simulink model "OutputCalibration"  (R2024b)
settings: Solver=FixedStepAuto  StartTime=0.0  StopTime=inf  FixedStep=1/200  RelTol=1e-3  EnableMultiTasking=on
libraries: mbedblockslib x3
settings Model: ExtModeTrigDuration=10  Creator=patri  LastModifiedBy=Jaylen
settings SolverCC: AutoInsertRateTranBlk=on
settings OptimizationCC: EnhancedBackFolding=on  PassReuseOutputArgsAs=Individual arguments  ZeroExternalMemoryAtStartup=off  ZeroInternalMemoryAtStartup=off  MaxStackSize=64  OptimizeBlockOrder=speed  DifferentSizesBufferReuse=on  OptimizationCustomize=off  EfficientTunableParamExpr=on
settings DebuggingCC: ParameterTunabilityLossMsg=error
settings HardwareCC: ProdBitPerPointer=32  ProdBitPerSizeT=32  ProdBitPerPtrDiffT=32  ProdLargestAtomicInteger=Long  ProdLargestAtomicFloat=Double  ProdWordSize=32  ProdLongLongMode=on  ProdHWDeviceType=ARM Compatible->ARM Cortex-M
settings SFSimCC: MATLABDynamicMemAlloc=off
settings RTWCC: Description=Embedded Coder  SystemTargetFile=ert.tlc  HardwareBoard=STM32 Nucleo F767ZI  TemplateMakefile=ert_default_tmf  Toolchain=GNU Tools for ARM Embedded Processors
settings CodeAppCC: ForceParamTrailComments=on  IgnoreCustomStorageClasses=off  OperatorAnnotations=on  SimulinkDataObjDesc=on  SFDataObjDesc=on  InsertBlockDesc=on
settings ERTTargetCC: ExtModeTransport=3  ExtModeStaticAlloc=on  ExtModeStaticAllocSize=10000  ExtModeMexFile=ext_xcp  ExtModeIntrfLevel=Level2 - Open  InlinedParameterPlacement=Hierarchical

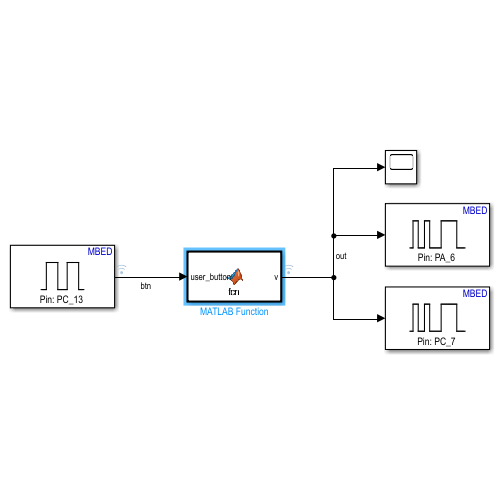
[thumbnail: Simulink's stored preview of the top-level diagram]
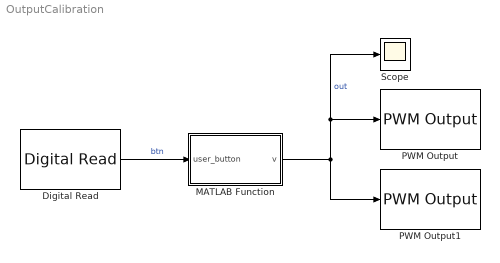
== system OutputCalibration ==
  Digital Read : mbedblockslib/Digital Read  Pin=PC_13  Direction=input  SampleTime=-1
      settings: LibrarySourceBlock=stmnucleorootlib/Common/Digital Read
  MATLAB Function : MATLAB Function  TreatAsAtomicUnit=on
  PWM Output : mbedblockslib/PWM Output  Pin=PA_6  EnableInputFrequency=off  InitialFrequency=10000  InitialDutyCycle=57.6  NotificationType=None
      settings: LibrarySourceBlock=stmnucleorootlib/Common/PWM Output
  PWM Output1 : mbedblockslib/PWM Output  Pin=PC_7  EnableInputFrequency=off  InitialFrequency=10000  InitialDutyCycle=57.6  NotificationType=None
      settings: LibrarySourceBlock=stmnucleorootlib/Common/PWM Output
  Scope : Scope
  wires:
  Digital Read/1 -> MATLAB Function/1(user_button)  "btn"
  MATLAB Function/1(v) -> PWM Output1/1, Scope/1, PWM Output/1  "out"

== matlab function OutputCalibration/MATLAB Function ==
  data: user_button input; v output
function v = fcn(user_button)

persistent m db i;
Fs = 200;

if isempty(m)
    m = 0;
    i = 0;
    db = 0;
end

if user_button == 1
    if db == 0
        db = 1;
        m = m + 10;
    end
end

if db == 1
    if i > 1*Fs
        db = 0;
        i = 0;
    else
        i = i + 1;
    end
end

v = m;
end
